simulink model "Controller"  (R2025b)
settings: Solver=VariableStepAuto  StartTime=0.0  StopTime=10.0  RelTol=1e-3
settings Model: Creator=bohdanusatov  LastModifiedBy=bohdanusatov

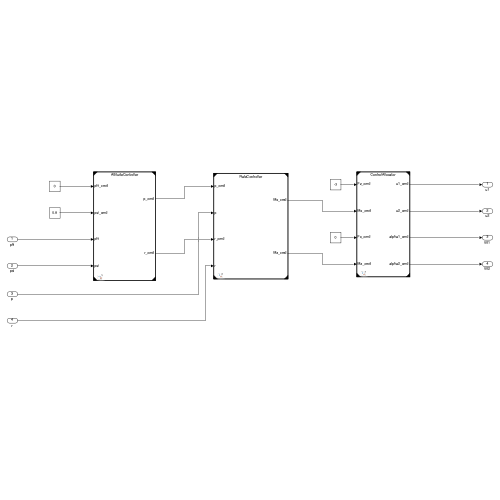
[thumbnail: Simulink's stored preview of the top-level diagram]
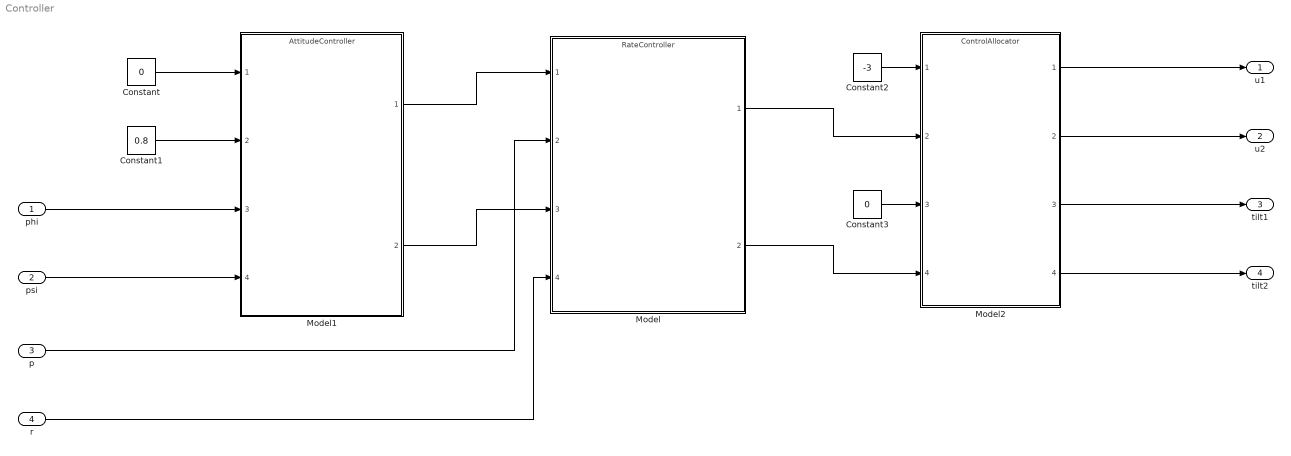
== system Controller ==
  phi : Inport
  psi : Inport  Port=2
  p : Inport  Port=3
  r : Inport  Port=4
  Constant : Constant  Value=0
  Constant1 : Constant  Value=0.8
  Constant2 : Constant  Value=-3
  Constant3 : Constant  Value=0
  Model : ModelReference  ModelNameDialog=RateController.slx  SimulationMode=Accelerator  ModelReferenceVersion=1.7
  Model1 : ModelReference  ModelNameDialog=AttitudeController.slx  SimulationMode=Accelerator  ModelReferenceVersion=1.5
  Model2 : ModelReference  ModelNameDialog=ControlAllocator.slx  SimulationMode=Accelerator  ModelReferenceVersion=1.4
  u1 : Outport
  u2 : Outport  Port=2
  tilt1 : Outport  Port=3
  tilt2 : Outport  Port=4
  wires:
  Model2/3 -> tilt1/1
  Model2/4 -> tilt2/1
  Model1/1 -> Model/1
  Model1/2 -> Model/3
  Model/2 -> Model2/4
  phi/1 -> Model1/3
  psi/1 -> Model1/4
  p/1 -> Model/2
  r/1 -> Model/4
  Constant1/1 -> Model1/2
  Constant/1 -> Model1/1
  Constant3/1 -> Model2/3
  Constant2/1 -> Model2/1
  Model2/1 -> u1/1
  Model2/2 -> u2/1
  Model/1 -> Model2/2
